simulink model "Grading_System"  (R2021a)
settings: Solver=FixedStepDiscrete  StartTime=0.0  StopTime=10.0  FixedStep=0.1  RelTol=1e-3  EnableMultiTasking=on
settings Model: Creator=alyma  LastModifiedBy=alyma
settings SolverCC: AlgebraicLoopSolver=TrustRegion  AutoInsertRateTranBlk=on
settings DataIOCC: LimitDataPoints=on
settings OptimizationCC: LifeSpan=inf
settings DebuggingCC: AllowSymbolicDim=off  SFUnexpectedBacktrackingDiag=warning  SFNoUnconditionalDefaultTransitionDiag=warning  SFExecutionAtInitializationDiag=none  ArithmeticOperatorsInVariantConditions=warning
settings SFSimCC: SimUseLocalCustomCode=off  CustomCodeUndefinedFunction=UseInterfaceOnly
settings RTWCC: RTWUseLocalCustomCode=off
settings CodeAppCC: StateflowObjectComments=on
settings GRTTargetCC: TargetLangStandard=C89/C90 (ANSI)
settings ConfigComp: CovMetricSettings=dw  CovSaveCumulativeToWorkspaceVar=on  CovSaveSingleToWorkspaceVar=on  CovExternalEMLEnable=off  CovSFcnEnable=off

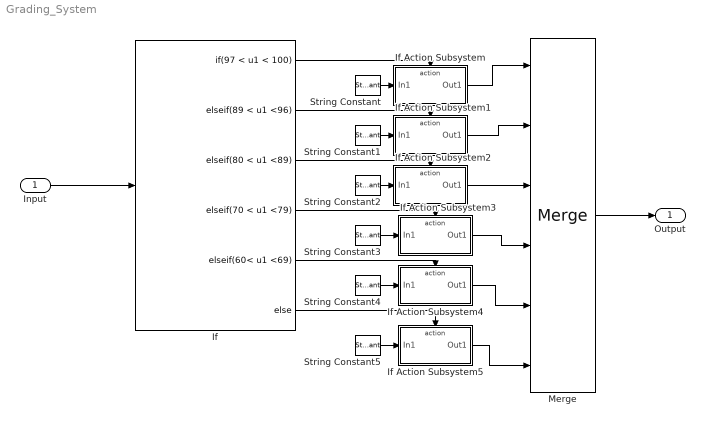
== system Grading_System ==
  Input : Inport
  If : If  IfExpression=97 < u1 < 100  ElseIfExpressions="89 < u1 <96 , 80 < u1 <89 ,  70 < u1 <79 , 60< u1 <69"
  If Action Subsystem : Subsystem  TreatAsAtomicUnit=on
  If Action Subsystem1 : Subsystem  TreatAsAtomicUnit=on
  If Action Subsystem2 : Subsystem  TreatAsAtomicUnit=on
  If Action Subsystem3 : Subsystem  TreatAsAtomicUnit=on
  If Action Subsystem4 : Subsystem  TreatAsAtomicUnit=on
  If Action Subsystem5 : Subsystem  TreatAsAtomicUnit=on
  Merge : Merge  Inputs=6
  String Constant : StringConstant  String="\"A+\""
  String Constant1 : StringConstant  String="\"A\""
  String Constant2 : StringConstant  String="\"B\""
  String Constant3 : StringConstant  String="\"C\""
  String Constant4 : StringConstant  String="\"D\""
  String Constant5 : StringConstant  String="\"F\""
  Output : Outport
  wires:
  Input/1 -> If/1
  If/1 -> If Action Subsystem/Action
  If/2 -> If Action Subsystem1/Action
  If/3 -> If Action Subsystem2/Action
  If/4 -> If Action Subsystem3/Action
  If/5 -> If Action Subsystem4/Action
  If/6 -> If Action Subsystem5/Action
  If Action Subsystem/1(Out1) -> Merge/1
  If Action Subsystem1/1(Out1) -> Merge/2
  If Action Subsystem2/1(Out1) -> Merge/3
  If Action Subsystem3/1(Out1) -> Merge/4
  If Action Subsystem4/1(Out1) -> Merge/5
  If Action Subsystem5/1(Out1) -> Merge/6
  Merge/1 -> Output/1
  String Constant/1 -> If Action Subsystem/1(In1)
  String Constant1/1 -> If Action Subsystem1/1(In1)
  String Constant2/1 -> If Action Subsystem2/1(In1)
  String Constant4/1 -> If Action Subsystem4/1(In1)
  String Constant3/1 -> If Action Subsystem3/1(In1)
  String Constant5/1 -> If Action Subsystem5/1(In1)

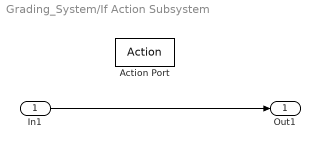
== system Grading_System/If Action Subsystem ==
  In1 : Inport
  Action Port : ActionPort  ActionPortLabel=if(97 < u1 < 100)
  Out1 : Outport
  wires:
  In1/1 -> Out1/1

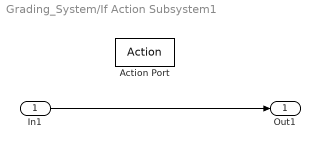
== system Grading_System/If Action Subsystem1 ==
  In1 : Inport
  Action Port : ActionPort  ActionPortLabel=elseif(89 < u1 <96 )
  Out1 : Outport
  wires:
  In1/1 -> Out1/1

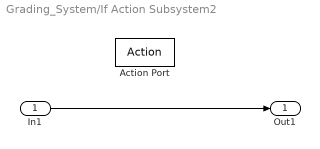
== system Grading_System/If Action Subsystem2 ==
  In1 : Inport
  Action Port : ActionPort  ActionPortLabel=elseif( 80 < u1 <89 )
  Out1 : Outport
  wires:
  In1/1 -> Out1/1

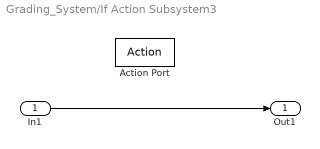
== system Grading_System/If Action Subsystem3 ==
  In1 : Inport
  Action Port : ActionPort  ActionPortLabel="elseif(  70 < u1 <79 )"
  Out1 : Outport
  wires:
  In1/1 -> Out1/1

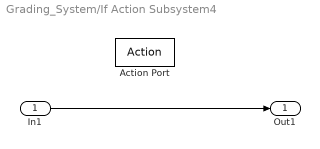
== system Grading_System/If Action Subsystem4 ==
  In1 : Inport
  Action Port : ActionPort  ActionPortLabel=elseif( 60< u1 <69)
  Out1 : Outport
  wires:
  In1/1 -> Out1/1

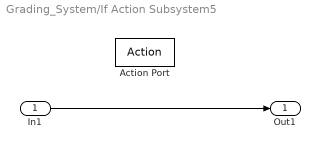
== system Grading_System/If Action Subsystem5 ==
  In1 : Inport
  Action Port : ActionPort  ActionPortLabel=else
  Out1 : Outport
  wires:
  In1/1 -> Out1/1
